simulink model "uart_test"  (R2023a)
settings: Solver=VariableStepAuto  StartTime=0.0  StopTime=inf  RelTol=1e-3
model workspace (MAT data in the model file):
  b_soc = Simulink.Parameter
  b_soc.DataType = 'auto'
  b_soc.Complexity = 'real'
  b_soc.Dimensions = [0 0]
  c_soc = Simulink.Parameter
  c_soc.DataType = 'auto'
  c_soc.Complexity = 'real'
  c_soc.Dimensions = [0 0]
  p_dmd = Simulink.Parameter
  p_dmd.DataType = 'auto'
  p_dmd.Complexity = 'real'
  p_dmd.Dimensions = [0 0]
values from neighbouring files (symbols this model uses):
  Bat_SOC = 0.96432    [tcp_double_test.m]    (also in tcp_socket_test.m = sprintf('; tcp_test.m = sprintf('; tcp_test_v2.m = sprintf('; tcp_test_v3.m = sprintf(')
  Cap_SOC = 0.83456    [tcp_double_test.m]    (also in tcp_socket_test.m = sprintf('; tcp_test.m = sprintf('; tcp_test_v2.m = sprintf('; tcp_test_v3.m = sprintf(')
  Pwr_Dmd = -0.57543    [tcp_double_test.m]    (also in tcp_socket_test.m = sprintf('; tcp_test.m = sprintf('; tcp_test_v2.m = sprintf('; tcp_test_v3.m = sprintf(')
undefined symbols (not defined in the file or in its folder): CR, LF
libraries: instrumentseriallib x3, instrumentlib x1
settings Model: Creator=antaeug  LastModifiedBy=tu101

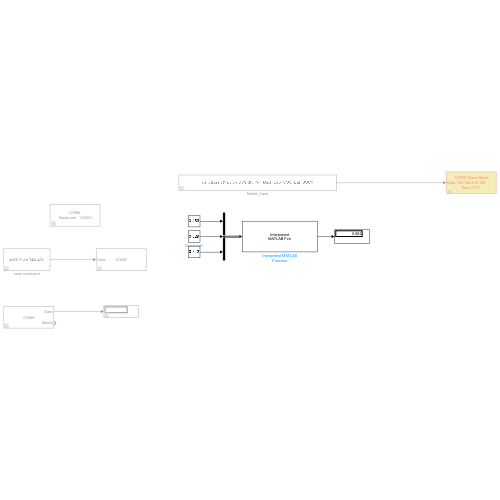
[thumbnail: Simulink's stored preview of the top-level diagram]
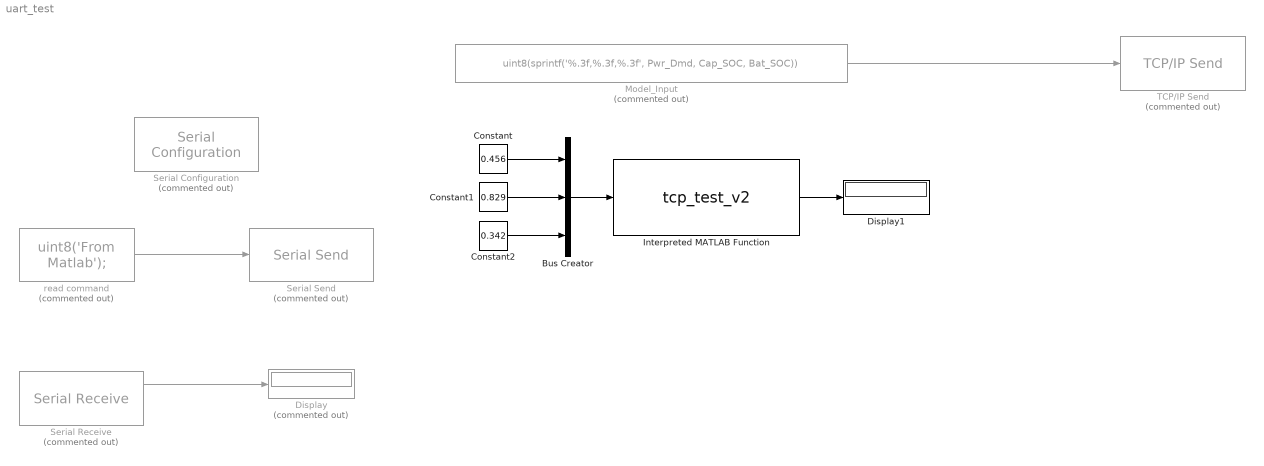
== system uart_test ==
  Bus Creator : BusCreator  Inputs=3
  Constant : Constant  Value=0.456
  Constant1 : Constant  Value=0.829
  Constant2 : Constant  Value=0.342
  Display : Display  Commented=on
      settings: Format=decimal (Stored Integer)
  Display1 : Display
  Interpreted MATLAB Function : MATLABFcn  MATLABFcn=tcp_test_v2
  Model_Input : Constant  Commented=on  Value=uint8(sprintf('%.3f,%.3f,%.3f', Pwr_Dmd, Cap_SOC, Bat_SOC))
  Serial Configuration : instrumentseriallib/Serial Configuration  Priority=-200000  Commented=on  PortSel=COM6  Port=COM6  ComPort=COM6  BaudRate=115200  DataBits=8  Parity=none  StopBits=1  ByteOrder=little-endian  FlowControl=none  Timeout=10  SimulateUsing=Interpreted execution  BlockInModel=on  aMode=1
  Serial Receive : instrumentseriallib/Serial Receive  Priority=1  Commented=on  PortSel=COM6  Port=COM6  ComPort=COM6  DataType=single  SaveDataType=uint8  ToggleHeader=off  Header=[]  ToggleTerminator=on  Terminator=CR/LF ('\r\n')  CustomTerminator=[]  InputFormat=Column major  ToggleDataSize=on  DataSize=[1 1]  EnableBlockingMode=off  ActionDataUnavailable=Output last received value  ActionWhenDataUnavailable=Output last received value  CustomValue=0  SampleTime=0.01  SimulateUsing=Interpreted execution  BlockInModel=on  aMode=1
  Serial Send : instrumentseriallib/Serial Send  Priority=1  Commented=on  PortSel=COM6  Port=COM6  ComPort=COM6  Header=[]  Terminator=CR/LF ('\r\n')  CustomTerminator=[]  EnableBlockingMode=on  SimulateUsing=Interpreted execution  BlockInModel=on  aMode=1
  TCP/IP Send : instrumentlib/TCP//IP Send  Commented=on  Host=192.168.219.100  Port=11111  ByteOrder=little-endian  EnableBlockingMode=on  Timeout=10  TransferDelay=on  SimulateUsing=Interpreted execution
  read command : Constant  Commented=on  Value=uint8('From Matlab');
  wires:
  read command/1 -> Serial Send/1
  Serial Receive/1 -> Display/1
  Model_Input/1 -> TCP/IP Send/1
  Constant/1 -> Bus Creator/1
  Constant1/1 -> Bus Creator/2
  Constant2/1 -> Bus Creator/3
  Bus Creator/1 -> Interpreted MATLAB Function/1
  Interpreted MATLAB Function/1 -> Display1/1
